simulink model "soccerVision_2017"  (R2017b)
settings: Solver=VariableStepAuto  StartTime=0.0  StopTime=inf  RelTol=1e-3
InitFcn:
  | visionConfiguration;
StartFcn:
  | visionConfiguration;
  | addpath('../soccer-strategy/');
  | connectRobot;
model workspace (MATLAB code in the model file):
  | visionConfiguration;
undefined symbols (not defined in the file or in its folder): gray, Rec, SDTV
libraries: robotlib x2, dspvision x1, visiongeotforms x1, visionconversions x1
settings Model: Creator=vuwij  LastModifiedBy=Farwa

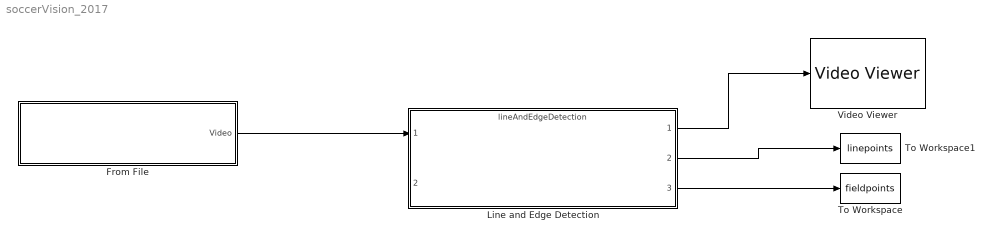
== system soccerVision_2017 ==
  From File : Subsystem  Variant=on  VariantControl=Variant1  OverrideUsingVariant=USE_GAZEBO==1
  Line and Edge Detection : ModelReference  ModelNameDialog=lineAndEdgeDetection  SimulationMode=Normal  ModelReferenceVersion=1.775
  To Workspace : ToWorkspace  VariableName=fieldpoints  SaveFormat=Timeseries  SampleTime=-1
  To Workspace1 : ToWorkspace  VariableName=linepoints  SaveFormat=Timeseries  SampleTime=-1
  Video Viewer : VideoViewer  colormapValue=gray(256)  FigPos=[42.3333333333333 740.666666666667 1214 563.333333333333]
  wires:
  Line and Edge Detection/3 -> To Workspace/1
  Line and Edge Detection/2 -> To Workspace1/1
  Line and Edge Detection/1 -> Video Viewer/1
  From File/1(" Video") -> Line and Edge Detection/1

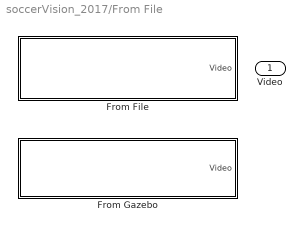
== system soccerVision_2017/From File ==
  From File : Subsystem  VariantControl=USE_GAZEBO==0
  From Gazebo : Subsystem  VariantControl=USE_GAZEBO==1
  " Video" : Outport

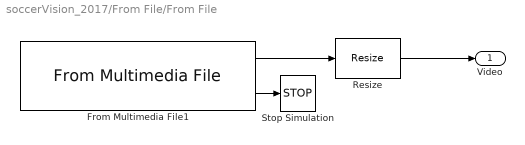
== system soccerVision_2017/From File/From File ==
  From Multimedia File1 : dspvision/From Multimedia File  inputFilename=C:\Users\Farwa\Documents\RoboSoccer\soccer-vision\media\videos\2.mp4  loop=on  numPlays=1  outputStreams=Video only  videoDataType=uint8  audioDataType=int16  inheritSampleTime=on  userDefinedSampleTime=0.1  noAudioOutput=off  isIntensityVideo=off  fourcc=Intensity  colorVideoFormat=One multidimensional signal  outputEOF=on  dataOrg=Column-major  audioFrameSize=1024  computeAudioFrameSize=off  outSamplingMode=Sample based
      settings: SourceProductBaseCode=VP
  Resize : visiongeotforms/Resize  specify=Number of output rows and columns  rfactor=[200 150]  outCols=25  outRows=25  outRowsCols=[480 640]  interp_method=Bilinear  antialias=on  useROI=off  roiFlag=off  prodOutputMode=Binary point scaling  prodOutputWordLength=32  prodOutputFracLength=10  roundingMode=Nearest  overflowMode=on
      settings: SourceProductName=Computer Vision System Toolbox  SourceProductBaseCode=VP
  Stop Simulation : Stop
  Video : Outport
  wires:
  From Multimedia File1/1 -> Resize/1
  From Multimedia File1/2 -> Stop Simulation/1
  Resize/1 -> Video/1

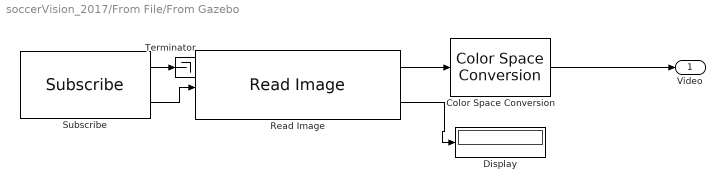
== system soccerVision_2017/From File/From Gazebo ==
  Color Space Conversion : visionconversions/Color Space  Conversion  conversion=Obsolete  conversionActive=R'G'B' to intensity  wp_str=D65  rec=Rec. 601 (SDTV)  sys=1125/60/2:1  imagePorts=One multidimensional signal
      settings: SourceProductName=Computer Vision System Toolbox
  Display : Display
  Read Image : robotlib/Read Image  SourceLibraryInfo=This block requires Robotics System Toolbox  MaximumImageSize=[480, 640]  ImageEncoding=rgb8  ShowAlphaOutput=off  ShowErrorCodeOutput=on  VariableSizeOutputs=off
      settings: SourceProductName=Robotics System Toolbox  SourceProductBaseCode=RO
  Subscribe : robotlib/Subscribe  SourceLibraryInfo=This block requires Robotics System Toolbox  topicSource=Select from ROS network  topic=/soccerbot/camera1/image_raw  messageType=sensor_msgs/Image  sampleTime=-1  messageQueueLength=1
      settings: SourceProductBaseCode=RO
  Terminator : Terminator
  Video : Outport
  wires:
  Subscribe/2 -> Read Image/1
  Read Image/1 -> Color Space Conversion/1
  Read Image/2 -> Display/1
  Subscribe/1 -> Terminator/1
  Color Space Conversion/1 -> Video/1
